simulink model "zad1"  (R2018b)
settings: Solver=VariableStepAuto  StartTime=0.0  StopTime=50  RelTol=1e-3
settings Model: Creator=krzys  LastModifiedBy=krzys

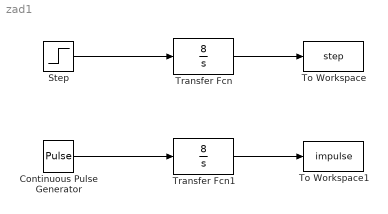
== system zad1 ==
  Continuous Pulse Generator : DiscretePulseGenerator  PulseType=Time based  Period=1  PulseWidth=50
  Step : Step  SampleTime=0
  To Workspace : ToWorkspace  VariableName=step  SaveFormat=Structure With Time  SampleTime=-1
  To Workspace1 : ToWorkspace  VariableName=impulse  SaveFormat=Structure With Time  SampleTime=-1
  Transfer Fcn : TransferFcn  Numerator=[8]  Denominator=[1 0]
  Transfer Fcn1 : TransferFcn  Numerator=[8]  Denominator=[1 0]
  wires:
  Transfer Fcn/1 -> To Workspace/1
  Step/1 -> Transfer Fcn/1
  Transfer Fcn1/1 -> To Workspace1/1
  Continuous Pulse Generator/1 -> Transfer Fcn1/1
